simulink model "SpeedControl"  (Simulink 10.0)
settings: Solver=ode1  StartTime=0.0  StopTime=inf  FixedStep=0.004  MaxStep=0.02  RelTol=1e-3  AbsTol=1e-6
libraries: mc9s12tool x1, simulink_extras x1
settings Model: Creator=fwornle  LastModifiedBy=bhisma  SimulationMode=external  ExtModeTrigDuration=2500
settings ConfigSet: Description=rtmc9s12target_R2009b
settings SolverCC: AutoScaleAbsTol=off
settings DataIOCC: SignalLoggingSaveFormat=ModelDataLogs  SaveOutput=off  SaveTime=off  SignalLoggingName=sigsOut
settings OptimizationCC: BlockReduction=off  BooleanDataType=off  ExpressionDepthLimit=2147483647  InitFltsAndDblsToZero=on  LifeSpan=1  EfficientTunableParamExpr=on
settings DebuggingCC: SaveWithParameterizedLinksMsg=none  SignalResolutionControl=TryResolveAllWithWarning  MultiTaskDSMMsg=warning  MultiTaskCondExecSysMsg=none  FcnCallInpInsideContextMsg=warning  StateNameClashWarn=warning
settings HardwareCC: ProdBitPerInt=16  ProdBitPerPointer=16  ProdBitPerSizeT=16  ProdBitPerPtrDiffT=16  ProdEndianess=BigEndian  ProdWordSize=16  ProdHWDeviceType=Motorola HC12
settings SFSimCC: MATLABDynamicMemAlloc=off
settings RTWCC: SystemTargetFile=mc9s12.tlc  GenerateMakefile=off  TemplateMakefile=mc9s12.tmf
settings CodeAppCC: IgnoreCustomStorageClasses=off  CustomSymbolStrType=$N$R$M  InternalIdentifier=Classic
settings STFCustomTargetCC: TargetFcnLib=ansi_tfl_tmw.mat  ModelReferenceCompliant=off  IncludeMdlTerminateFcn=off  ERTCustomFileBanners=on  SupportNonInlinedSFcns=off  RemoveResetFunc=on  MATLABClassNameForMDSCustomization=Simulink.SoftwareTarget.ERTCustomization  CPPClassGenCompliant=on  SystemTargetFile=mc9s12.tlc
settings ERTTargetCC: TargetFcnLib=ansi_tfl_tmw.mat  MultiwordLength=2048  ModelReferenceCompliant=off  ParMdlRefBuildCompliant=off  CompOptLevelCompliant=off  ConcurrentExecutionCompliant=off  IncludeMdlTerminateFcn=off  CombineOutputUpdateFcns=off  SupportContinuousTime=on  ModelStepFunctionPrototypeControlCompliant=off  GRTInterface=on  UseToolchainInfoCompliant=off  ExtMode=on  ExtModeMexFile=ext_serial_mc9s12_comm  ExtModeMexArgs=1,2,115200  ERTCustomFileTemplate=mc9s12_file_process.tlc  ConvertIfToSwitch=off  SuppressUnreachableDefaultCases=off
settings CustomProperty: DataType=RTWOptions_EnumType_C__Users_fw__SVN_rtmc9s12-target_trunk_rtmc9s12_CW_R2009b_bin_mc9s12_1mc9s12_TargetBoard  Value=Dragon12Plus
settings EnumStrPairs: String=Dragon12
settings ConfigComp: CovExternalEMLEnable=off

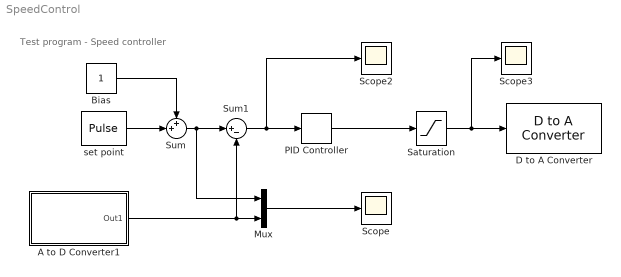
== system SpeedControl ==
  note: Test program - Speed controller
  A to D Converter1 : Subsystem  Tag=mcTarget_adc  mask{bank=0, channels=3, use10bits=10 bits, normalize=max. output:  5, sampletime=0.004}
      mask prompts: bank "ADC bank"; channels "Channels ( 0 - 7 )"; use10bits "ADC resolution"; normalize "Normalization"; sampletime "Sample time"
      mask init:
      | [channelsStr, firstChannel, numChannels] = mbc_adcinput(channels);
      mask Help: web('adc_sfcn_9S12.html');
      mask TypeOptions bank: 0 | 1
      mask TypeOptions use10bits: 10 bits | 8 bits
      mask TypeOptions normalize: raw values | max. output:  1 | max. output:  5
      mask Display: disp(['A to D Converter\n' channelsStr])
  Bias : Constant
  D to A Converter : mc9s12tool/D to A Converter  Tag=mcTarget_dac  SystemSampleTime=-1  sampletime=0.004  dac_channel=1  Vsat=5
  Mux : Mux  Inputs=2
  PID Controller : simulink_extras/Additional Linear/PID Controller  SystemSampleTime=-1  P=1  I=0  D=0
      settings: SourceProductName=Simulink  SourceProductBaseCode=SL
  Saturation : Saturate  UpperLimit=5  LowerLimit=0
  Scope : Scope
  Scope2 : Scope
  Scope3 : Scope
  Sum : Sum  Inputs=++|  SaturateOnIntegerOverflow=on
  Sum1 : Sum  Inputs=|+-  SaturateOnIntegerOverflow=on
  set point : DiscretePulseGenerator  PulseType=Time based  Amplitude=3  PulseWidth=50
  wires:
  Saturation/1 -> Scope3/1, D to A Converter/1
  A to D Converter1/1(Out1) -> Mux/2, Sum1/2
  PID Controller/1 -> Saturation/1
  Mux/1 -> Scope/1
  Bias/1 -> Sum/1
  set point/1 -> Sum/2
  Sum/1 -> Sum1/1, Mux/1
  Sum1/1 -> PID Controller/1, Scope2/1

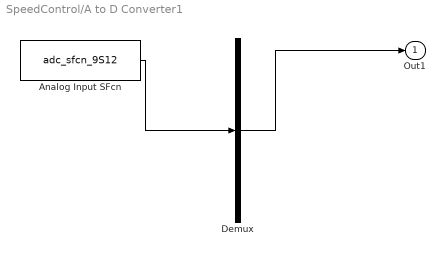
== system SpeedControl/A to D Converter1 ==
  Analog Input SFcn : S-Function  Tag=mcTarget_adc  FunctionName=adc_sfcn_9S12  Parameters=bank-1, firstChannel, numChannels, use10bits-1, normalize, sampletime  SFunctionDeploymentMode=off  EnableBusSupport=off
  Demux : Demux  Outputs=1
  Out1 : Outport
  wires:
  Analog Input SFcn/1 -> Demux/1
  Demux/1 -> Out1/1
